simulink model "ground_state_ridgid"  (R2017b)
settings: Solver=VariableStepAuto  StartTime=0.0  StopTime=10  RelTol=1e-3
undefined symbols (not defined in the file or in its folder): refo
settings Model: Creator=benma  LastModifiedBy=benma

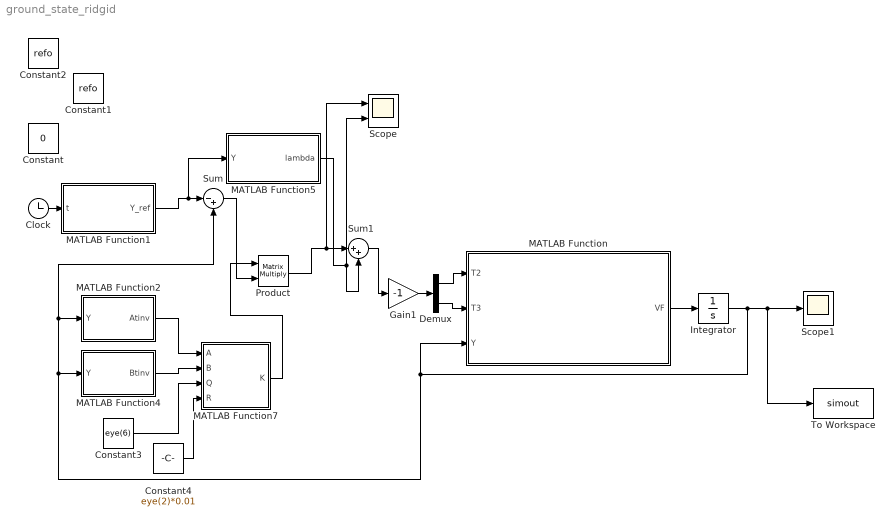
== system ground_state_ridgid ==
  Clock : Clock
  Constant : Constant  Value=0
  Constant1 : Constant  Value=refo
  Constant2 : Constant  Value=refo
  Constant3 : Constant  Value=eye(6)
  Constant4 : Constant  Value=eye(2)*0.01
  Demux : Demux  Outputs=2
  Gain1 : Gain  Gain=-1
  Integrator : Integrator  InitialCondition=refo
  MATLAB Function : MATLAB Function  TreatAsAtomicUnit=on
  MATLAB Function1 : MATLAB Function  TreatAsAtomicUnit=on
  MATLAB Function2 : MATLAB Function  TreatAsAtomicUnit=on
  MATLAB Function4 : MATLAB Function  TreatAsAtomicUnit=on
  MATLAB Function5 : MATLAB Function  TreatAsAtomicUnit=on
  MATLAB Function7 : MATLAB Function  TreatAsAtomicUnit=on
  Product : Product  Multiplication=Matrix(*)
  Scope : Scope  NumInputPorts=2
  Scope1 : Scope
  Sum : Sum  Inputs=|-+
  Sum1 : Sum  Inputs=|++
  To Workspace : ToWorkspace  VariableName=simout  SaveFormat=Timeseries  SampleTime=-1
  wires:
  MATLAB Function/1(VF) -> Integrator/1
  Gain1/1 -> Demux/1
  Demux/1 -> MATLAB Function/1(T2)
  Demux/2 -> MATLAB Function/2(T3)
  MATLAB Function5/1(lambda) -> Sum1/2, Scope/2
  Sum1/1 -> Gain1/1
  Clock/1 -> MATLAB Function1/1(t)
  MATLAB Function1/1(Y_ref) -> MATLAB Function5/1(Y), Sum/1
  Integrator/1 -> To Workspace/1, Scope1/1, MATLAB Function/3(Y), MATLAB Function4/1(Y), MATLAB Function2/1(Y), Sum/2
  MATLAB Function2/1(Atinv) -> MATLAB Function7/1(A)
  MATLAB Function4/1(Btinv) -> MATLAB Function7/2(B)
  Constant3/1 -> MATLAB Function7/3(Q)
  Constant4/1 -> MATLAB Function7/4(R)
  Product/1 -> Scope/1, Sum1/1
  Sum/1 -> Product/2
  MATLAB Function7/1(K) -> Product/1

== matlab function ground_state_ridgid/MATLAB Function ==
  data: T2 input; VF output; T3 input; Y input
function VF = threedof_ground(T2,T3,Y)
%THREEDOF_GROUND
%    VF = THREEDOF_GROUND(T2,T3,Y)

%    This function was generated by the Symbolic Math Toolbox version 8.0.
%    23-Nov-2018 17:29:58

t2 = Y(2);
t3 = t2.*2.0;
t4 = Y(3);
t5 = t4.*2.0;
t6 = Y(1);
t7 = Y(4);
t8 = t7.^2;
t9 = t2-t4;
t10 = sin(t9);
t11 = Y(5);
t12 = Y(6);
t13 = t2+t5;
t14 = sin(t13);
t15 = t11.^2;
t16 = cos(t5);
t17 = cos(t13);
t18 = t3+t5;
t19 = sin(t2);
t20 = t2+t4;
t21 = sin(t20);
t22 = t12.^2;
t23 = cos(t2);
t24 = cos(t3);
t25 = t24.*8.1e1;
t26 = t16.*4.5e1;
t27 = cos(t18);
t66 = t27.*9.0;
t28 = t25+t26-t66-1.69e2;
t29 = 1.0./t28;
t30 = cos(t6);
t31 = t3+t6;
t32 = cos(t31);
t33 = t32.*1.32435e4;
t34 = -t5+t6;
t35 = cos(t34);
t36 = t35.*4.4145e3;
t37 = t5+t6;
t38 = cos(t37);
t39 = t38.*4.4145e3;
t40 = t3+t5+t6;
t41 = cos(t40);
t42 = sin(t3);
t43 = sin(t5);
t44 = t8.*t10.*4.5e2;
t45 = t10.*t15.*4.5e2;
t46 = t10.*t22.*4.5e2;
t47 = t3+t4;
t48 = sin(t47);
t49 = cos(t9);
t50 = T3.*t17.*9.0e2;
t51 = sin(t18);
t52 = t15.*t19.*2.25e3;
t53 = sin(t4);
t54 = t8.*t21.*2.5e2;
t55 = t15.*t21.*2.5e2;
t56 = t21.*t22.*2.5e2;
t57 = cos(t20);
t58 = T3.*t57.*2.1e3;
t59 = t7.*t11.*t21.*5.0e2;
t60 = t7.*t12.*t21.*5.0e2;
t61 = t11.*t12.*t21.*5.0e2;
t62 = t7.*t10.*t11.*9.0e2;
t63 = t7.*t10.*t12.*9.0e2;
t64 = t10.*t11.*t12.*9.0e2;
t65 = t7.*t11.*t19.*4.5e3;
t67 = t2+t6;
t68 = cos(t67);
t69 = t68.*2.20725e4;
t70 = t2+t5+t6;
t71 = cos(t70);
t72 = -t2+t6;
t73 = cos(t72);
t74 = t2+t5-t6;
t75 = cos(t74);
t76 = t75.*4.4145e3;
t77 = t8.*t42.*1.35e3;
t78 = t15.*t42.*1.35e3;
t79 = t22.*t48.*4.5e2;
t80 = cos(t47);
t81 = T3.*t27.*9.0e2;
t82 = T2.*t23.*2.7e3;
t83 = cos(t4);
t84 = t7.*t11.*t42.*2.7e3;
t85 = t7.*t12.*t48.*9.0e2;
t86 = t11.*t12.*t48.*9.0e2;
VF = [t7;t11;t12;t29.*(T2.*2.3e3-t30.*3.1392e4+t33+t36+t39-t41.*1.4715e3+t44+t45+t46+t50+t52+t54+t55+t56+t58+t59+t60+t61+t62+t63+t64+t65+t77+t82-T2.*t16.*9.0e2-T2.*t17.*9.0e2-T3.*t23.*2.7e3-T3.*t49.*2.7e3-t8.*t14.*1.5e2+t8.*t19.*2.25e3-t14.*t15.*1.5e2-t8.*t51.*1.5e2-t7.*t11.*t14.*3.0e2).*(-3.0./5.0e1);t29.*(T2.*7.0e3-T3.*4.7e3-t30.*3.1392e4+t33+t36+t39-t41.*1.4715e3+t44+t45+t46+t50+t52+t54+t55+t56+t58+t59+t60+t61+t62+t63+t64+t65+t69-t71.*2.943e3-t73.*2.6487e4+t76+t78+t79+t81+t84+t85+t86-T2.*t16.*9.0e2-T2.*t17.*1.8e3+T2.*t23.*5.4e3-T3.*t23.*2.7e3-T2.*t27.*9.0e2-T3.*t49.*2.7e3+T3.*t80.*2.7e3-T3.*t83.*5.7e3-t8.*t14.*9.0e2+t8.*t19.*7.2e3-t14.*t15.*1.5e2+t8.*t42.*2.7e3-t8.*t43.*7.5e2+t8.*t48.*4.5e2-t15.*t43.*7.5e2-t8.*t51.*1.5e2-t8.*t53.*1.45e3+t15.*t48.*4.5e2-t15.*t53.*1.45e3-t22.*t53.*1.45e3-t7.*t11.*t14.*3.0e2-t7.*t11.*t43.*1.5e3+t7.*t11.*t48.*9.0e2-t7.*t11.*t53.*2.9e3-t7.*t12.*t53.*2.9e3-t11.*t12.*t53.*2.9e3).*(3.0./5.0e1);t29.*(T2.*4.7e3-T3.*1.9e4+t69-t71.*2.943e3-t73.*2.6487e4+t76+t77+t78+t79+t81+t82+t84+t85+t86-cos(t2+t4+t6).*2.4525e3+cos(t2+t4-t6).*5.886e3+cos(t2-t4+t6).*8.829e3-cos(-t2+t4+t6).*1.32435e4-T2.*t17.*9.0e2+T3.*t24.*8.1e3-T2.*t27.*9.0e2+T2.*t49.*2.7e3-T2.*t57.*2.1e3-T2.*t80.*2.7e3+T3.*t80.*5.4e3+T2.*t83.*5.7e3-T3.*t83.*1.14e4+t8.*t10.*2.25e3-t8.*t14.*7.5e2+t8.*t19.*4.95e3-t8.*t21.*8.5e2-t8.*t43.*1.5e3+t8.*t48.*9.0e2-t15.*t43.*1.5e3+t8.*t51.*1.5e2-t8.*t53.*5.0e3+t15.*t48.*9.0e2-t22.*t43.*7.5e2+t15.*t51.*1.5e2-t15.*t53.*5.0e3+t22.*t51.*1.5e2-t22.*t53.*1.45e3-t7.*t11.*t43.*3.0e3-t7.*t12.*t43.*1.5e3+t7.*t11.*t48.*1.8e3-t11.*t12.*t43.*1.5e3+t7.*t11.*t51.*3.0e2+t7.*t12.*t51.*3.0e2-t7.*t11.*t53.*1.0e4-t7.*t12.*t53.*2.9e3+t11.*t12.*t51.*3.0e2-t11.*t12.*t53.*2.9e3).*(-3.0./5.0e1)];

== matlab function ground_state_ridgid/MATLAB Function1 ==
  data: t input; Y_ref output
function Y_ref = Reference(t)
%REFERENCE
%    Y_REF = REFERENCE(T)

%    This function was generated by the Symbolic Math Toolbox version 8.0.
%    15-Dec-2018 14:08:43

t2 = t.^2;
t3 = exp(t2);
t4 = 1.0./t3.^(1.0./3.0);
t5 = exp(-2.5e1./3.0);
t6 = exp(t);
t7 = t6.^(1.0e1./3.0);
t8 = t4.*t5.*t7.*pi.*(1.0./2.0);
t9 = cos(t8);
t10 = sin(t8);
t11 = t-5.0;
t12 = t11.^2;
t26 = t12.*(1.0./3.0);
t13 = exp(-t26);
t14 = t9.*4.0;
t15 = t9.^2;
t16 = t10.^2;
t17 = t14+t15+t16+4.0;
t18 = sqrt(t17);
t19 = t10+t18;
t20 = t9+2.0;
t21 = 1.0./t20;
t22 = t4.*t5.*t6.^(1.0e1./3.0).*pi.*(5.0./3.0);
t25 = t.*t4.*t5.*t7.*pi.*(1.0./3.0);
t23 = t22-t25;
t24 = 1.0./t20.^2;
t27 = t.*(2.0./3.0);
t28 = t27-1.0e1./3.0;
t29 = t13.*t28.*pi.*(1.0./2.0);
Y_ref = [atan(t19.*t21).*2.0;t13.*pi.*(-1.0./2.0);t13.*pi.*(1.0./2.0);(t21.*(t9.*t23-t10.*1.0./sqrt(t17).*t23.*2.0).*2.0+t10.*t19.*t23.*t24.*2.0)./(t19.^2.*t24+1.0);t29;-t29];

== matlab function ground_state_ridgid/MATLAB Function2 ==
  data: Y input; Atinv output
function Atinv = LinA(Y)
%LINA
%    ATINV = LINA(Y)

%    This function was generated by the Symbolic Math Toolbox version 8.0.
%    15-Dec-2018 02:05:19

t2 = Y(2);
t3 = t2.*2.0;
t4 = Y(3);
t5 = t4.*2.0;
t6 = Y(1);
t7 = cos(t3);
t8 = t7.*8.1e1;
t9 = cos(t5);
t10 = t9.*4.5e1;
t11 = t3+t5;
t12 = cos(t11);
t152 = t12.*9.0;
t13 = t8+t10-t152-1.69e2;
t14 = 1.0./t13;
t15 = t3+t6;
t16 = sin(t15);
t17 = t3+t5+t6;
t18 = sin(t17);
t19 = Y(4);
t20 = t2-t4;
t21 = cos(t20);
t22 = Y(5);
t23 = t19.^2;
t24 = Y(6);
t25 = t2+t5;
t26 = cos(t25);
t27 = t22.^2;
t28 = cos(t2);
t29 = t2+t4;
t30 = cos(t29);
t31 = t24.^2;
t32 = sin(t5);
t33 = sin(t20);
t34 = t3+t4;
t35 = sin(t34);
t36 = sin(t25);
t37 = sin(t11);
t38 = sin(t4);
t39 = sin(t29);
t40 = sin(t2);
t41 = t28.*3.0;
t42 = cos(t4);
t43 = t30+t41+t42+4.0;
t44 = 1.0./t43;
t45 = cos(t6);
t46 = t2+t6;
t47 = cos(t46);
t48 = t4+t6;
t49 = cos(t48);
t50 = t2+t4-t6;
t51 = cos(t50);
t52 = t3+t4+t6;
t53 = cos(t52);
t54 = -t4+t6;
t55 = cos(t54);
t56 = cos(t17);
t57 = t56.*1.4715e3;
t58 = t2+t4+t6;
t59 = cos(t58);
t60 = sin(t3);
t61 = t23.*t37.*3.0e2;
t62 = t27.*t37.*1.5e2;
t63 = t31.*t37.*1.5e2;
t64 = t23.*t39.*3.3e3;
t65 = t19.*t22.*t37.*3.0e2;
t66 = t19.*t24.*t37.*3.0e2;
t67 = t22.*t24.*t37.*3.0e2;
t68 = t49.*1.4715e3;
t69 = t2-t4+t6;
t70 = cos(t69);
t71 = t53.*4.4145e3;
t72 = t2+t5+t6;
t73 = cos(t72);
t74 = t73.*1.4715e3;
t75 = t59.*9.81e3;
t76 = t23.*t32.*3.0e2;
t77 = t27.*t32.*3.0e2;
t78 = t31.*t32.*1.5e2;
t79 = t23.*t33.*9.0e2;
t80 = t23.*t35.*9.0e2;
t81 = t23.*t36.*6.0e2;
t82 = t27.*t35.*4.5e2;
t83 = t27.*t36.*4.5e2;
t84 = t31.*t36.*3.0e2;
t85 = t27.*t40.*4.5e2;
t86 = t23.*t38.*3.3e3;
t87 = t27.*t38.*1.95e3;
t88 = t31.*t38.*2.0e2;
t89 = t27.*t39.*1.55e3;
t90 = t31.*t39.*2.0e2;
t91 = t19.*t22.*t39.*3.1e3;
t92 = t19.*t24.*t39.*4.0e2;
t93 = t22.*t24.*t39.*4.0e2;
t94 = t19.*t22.*t32.*6.0e2;
t95 = t19.*t24.*t32.*3.0e2;
t96 = t22.*t24.*t32.*3.0e2;
t97 = t19.*t22.*t35.*9.0e2;
t98 = t19.*t22.*t36.*9.0e2;
t99 = t19.*t24.*t36.*6.0e2;
t100 = t22.*t24.*t36.*6.0e2;
t101 = t19.*t22.*t40.*9.0e2;
t102 = t19.*t22.*t38.*3.9e3;
t103 = t19.*t24.*t38.*4.0e2;
t104 = t22.*t24.*t38.*4.0e2;
t107 = t51.*7.3575e3;
t145 = t45.*8.3385e3;
t146 = t47.*4.4145e3;
t147 = t70.*4.4145e3;
t148 = t55.*1.1772e4;
t149 = t27.*t33.*4.5e2;
t150 = t19.*t22.*t33.*9.0e2;
t105 = t57+t61+t62+t63+t64+t65+t66+t67+t68+t71+t74+t75+t76+t77+t78-t79+t80+t81+t82+t83+t84+t85+t86+t87+t88+t89+t90+t91+t92+t93+t94+t95+t96+t97+t98+t99+t100+t101+t102+t103+t104-t107-t145-t146-t147-t148-t149-t150;
t106 = t47.*1.91295e4;
t108 = t53.*8.829e3;
t109 = -t2+t6;
t110 = cos(t109);
t111 = cos(t15);
t112 = t111.*1.32435e4;
t113 = t59.*6.3765e3;
t114 = t23.*t60.*2.7e3;
t115 = t27.*t60.*1.35e3;
t116 = t27.*t33.*9.0e2;
t117 = t23.*t35.*1.8e3;
t118 = t23.*t36.*3.0e2;
t119 = t31.*t33.*4.5e2;
t120 = t27.*t35.*9.0e2;
t121 = t27.*t36.*3.0e2;
t122 = t31.*t35.*4.5e2;
t123 = t31.*t36.*1.5e2;
t124 = t23.*t40.*7.5e3;
t125 = t27.*t40.*3.3e3;
t126 = t31.*t40.*4.5e2;
t127 = t27.*t39.*1.9e3;
t128 = t31.*t39.*5.5e2;
t129 = t19.*t22.*t39.*3.8e3;
t130 = t19.*t24.*t39.*1.1e3;
t131 = t22.*t24.*t39.*1.1e3;
t132 = t19.*t22.*t60.*2.7e3;
t133 = t19.*t22.*t33.*1.8e3;
t134 = t19.*t24.*t33.*9.0e2;
t135 = t19.*t22.*t35.*1.8e3;
t136 = t19.*t22.*t36.*6.0e2;
t137 = t22.*t24.*t33.*9.0e2;
t138 = t19.*t24.*t35.*9.0e2;
t139 = t19.*t24.*t36.*3.0e2;
t140 = t22.*t24.*t35.*9.0e2;
t141 = t22.*t24.*t36.*3.0e2;
t142 = t19.*t22.*t40.*6.6e3;
t143 = t19.*t24.*t40.*9.0e2;
t144 = t22.*t24.*t40.*9.0e2;
t155 = t45.*3.4335e4;
t156 = t49.*1.03005e4;
t157 = t110.*2.20725e4;
t158 = t55.*1.03005e4;
t159 = t31.*t38.*9.5e2;
t160 = t19.*t24.*t38.*1.9e3;
t161 = t22.*t24.*t38.*1.9e3;
t151 = t57+t61+t62+t63+t64+t65+t66+t67+t79+t106-t107+t108+t112+t113+t114+t115+t116+t117+t118+t119+t120+t121+t122+t123+t124+t125+t126+t127+t128+t129+t130+t131+t132+t133+t134+t135+t136+t137+t138+t139+t140+t141+t142+t143+t144-t155-t156-t157-t158-t159-t160-t161;
t153 = -t5+t6;
t154 = t5+t6;
t162 = sin(t153);
t163 = sin(t154);
t164 = t18.*2.943e3;
t165 = t21.*t23.*4.5e2;
t166 = t21.*t27.*4.5e2;
t167 = t21.*t31.*4.5e2;
t168 = t23.*t30.*2.5e2;
t169 = t27.*t30.*2.5e2;
t170 = t30.*t31.*2.5e2;
t171 = t19.*t22.*t30.*5.0e2;
t172 = t19.*t24.*t30.*5.0e2;
t173 = t22.*t24.*t30.*5.0e2;
t174 = t39.*t44.*t105.*(7.0./4.0);
t175 = t19.*t21.*t22.*9.0e2;
t176 = t19.*t21.*t24.*9.0e2;
t177 = t21.*t22.*t24.*9.0e2;
t178 = t37.*1.8e1;
t179 = 1.0./t13.^2;
t180 = cos(t153);
t181 = t180.*4.4145e3;
t182 = cos(t154);
t183 = t182.*4.4145e3;
t184 = t23.*t60.*1.35e3;
t185 = t23.*t33.*4.5e2;
t186 = t23.*t40.*2.25e3;
t187 = t27.*t40.*2.25e3;
t188 = t23.*t39.*2.5e2;
t189 = t27.*t39.*2.5e2;
t190 = t31.*t39.*2.5e2;
t191 = t9.*t44.*t151.*(3.0./4.0);
t192 = t19.*t22.*t39.*5.0e2;
t193 = t19.*t24.*t39.*5.0e2;
t194 = t22.*t24.*t39.*5.0e2;
t195 = t26.*t44.*t151.*(3.0./4.0);
t196 = t21.*t44.*t105.*(9.0./4.0);
t197 = t28.*t44.*t105.*(9.0./4.0);
t198 = t19.*t22.*t40.*4.5e3;
t228 = t45.*3.1392e4;
t229 = t27.*t36.*1.5e2;
t230 = t23.*t37.*1.5e2;
t231 = t26.*t44.*t105.*(3.0./4.0);
t232 = t19.*t22.*t36.*3.0e2;
t233 = t30.*t44.*t105.*(7.0./4.0);
t275 = t28.*t44.*t151.*(9.0./4.0);
t199 = -t57+t112+t119+t134+t137+t149+t150+t181+t183+t184+t185+t186+t187+t188+t189+t190+t191+t192+t193+t194+t195+t196+t197+t198-t228-t229-t230-t231-t232-t233-t275-t23.*t36.*1.5e2-t44.*t151.*(2.3e1./1.2e1);
t200 = t19.*t40.*4.5e3;
t201 = t22.*t40.*4.5e3;
t202 = t19.*t39.*5.0e2;
t203 = t22.*t39.*5.0e2;
t204 = t24.*t39.*5.0e2;
t205 = t19.*t33.*9.0e2;
t206 = t22.*t33.*9.0e2;
t207 = t24.*t33.*9.0e2;
t208 = sin(t6);
t209 = t16.*1.32435e4;
t210 = t162.*4.4145e3;
t211 = t163.*4.4145e3;
t212 = sin(t46);
t213 = sin(t72);
t214 = t213.*2.943e3;
t215 = sin(t109);
t216 = t215.*2.6487e4;
t217 = t2+t5-t6;
t218 = sin(t217);
t219 = t218.*4.4145e3;
t220 = cos(t34);
t221 = t12.*t23.*3.0e2;
t222 = t27.*t28.*2.25e3;
t223 = t36.*t44.*t151.*(3.0./2.0);
t224 = t36.*t44.*t105.*(3.0./4.0);
t225 = t19.*t22.*t28.*4.5e3;
t226 = t60.*1.62e2;
t227 = t178-t226;
t234 = t163.*8.829e3;
t235 = t26.*t27.*3.0e2;
t236 = t32.*t44.*t151.*(3.0./2.0);
t237 = t19.*t22.*t26.*6.0e2;
t238 = t37.*t44.*t105.*(3.0./2.0);
t239 = t32.*9.0e1;
t240 = t178-t239;
t241 = t47.*2.20725e4;
t242 = cos(t217);
t243 = t242.*4.4145e3;
t244 = t23.*t35.*4.5e2;
t245 = t23.*t40.*7.2e3;
t246 = t44.*t105.*(4.7e1./1.2e1);
t247 = t26.*t44.*t151.*(3.0./2.0);
t248 = t12.*t44.*t151.*(3.0./4.0);
t249 = t42.*t44.*t105.*(1.9e1./4.0);
t272 = t73.*2.943e3;
t273 = t110.*2.6487e4;
t274 = t31.*t38.*1.45e3;
t276 = t12.*t44.*t105.*(3.0./4.0);
t277 = t19.*t24.*t38.*2.9e3;
t278 = t22.*t24.*t38.*2.9e3;
t250 = -t57+t82+t97+t112+t114+t115+t119+t122+t132+t134+t137+t138+t140+t149+t150+t181+t183+t185+t187+t188+t189+t190+t191+t192+t193+t194+t196+t197+t198-t228-t229-t230-t231-t232-t233+t241+t243+t244+t245+t246+t247+t248+t249-t272-t273-t274-t276-t277-t278-t23.*t32.*7.5e2-t23.*t36.*9.0e2-t27.*t32.*7.5e2-t23.*t38.*1.45e3-t27.*t38.*1.45e3-t44.*t151.*(3.5e1./6.0)-t19.*t22.*t32.*1.5e3-t19.*t22.*t38.*2.9e3-t28.*t44.*t151.*(9.0./2.0)-t44.*t105.*t220.*(9.0./4.0);
t251 = t19.*t60.*2.7e3;
t252 = t22.*t60.*2.7e3;
t253 = t19.*t35.*9.0e2;
t254 = t22.*t35.*9.0e2;
t255 = t24.*t35.*9.0e2;
t256 = sin(t50);
t257 = t256.*5.886e3;
t258 = -t2+t4+t6;
t259 = sin(t258);
t260 = t259.*1.32435e4;
t261 = sin(t69);
t262 = sin(t58);
t263 = t262.*2.4525e3;
t264 = t31.*t220.*9.0e2;
t265 = t7.*t23.*2.7e3;
t266 = t7.*t27.*2.7e3;
t267 = t7.*t19.*t22.*5.4e3;
t268 = t19.*t24.*t220.*1.8e3;
t269 = t22.*t24.*t220.*1.8e3;
t270 = t37.*t44.*t151.*(3.0./2.0);
t271 = t40.*t44.*t151.*(9.0./4.0);
t279 = t218.*8.829e3;
t280 = t21.*t23.*2.25e3;
t281 = t23.*t220.*9.0e2;
t282 = t27.*t220.*9.0e2;
t283 = t12.*t27.*3.0e2;
t284 = t12.*t31.*3.0e2;
t285 = t31.*t42.*1.45e3;
t286 = t33.*t44.*t151.*(9.0./4.0);
t287 = t19.*t22.*t220.*1.8e3;
t288 = t35.*t44.*t105.*(9.0./2.0);
t289 = t12.*t19.*t22.*6.0e2;
t290 = t12.*t19.*t24.*6.0e2;
t291 = t12.*t22.*t24.*6.0e2;
t292 = t19.*t24.*t42.*2.9e3;
t293 = t22.*t24.*t42.*2.9e3;
t294 = t51.*5.886e3;
t295 = cos(t258);
t296 = t70.*8.829e3;
t297 = t23.*t33.*2.25e3;
t298 = t23.*t40.*4.95e3;
t299 = t44.*t105.*(9.5e1./6.0);
t300 = t44.*t151.*t220.*(9.0./4.0);
t301 = t30.*t44.*t151.*(7.0./4.0);
t302 = t42.*t44.*t105.*(1.9e1./2.0);
t303 = t59.*(-2.4525e3)+t62+t63+t65+t66+t67+t80+t115+t120+t122+t132+t135+t138+t140+t184+t195+t230+t241+t243+t248-t272-t273-t274-t275-t276-t277-t278+t294-t295.*1.32435e4+t296+t297+t298+t299+t300+t301+t302-t23.*t32.*1.5e3-t23.*t36.*7.5e2-t27.*t32.*1.5e3-t23.*t38.*5.0e3-t23.*t39.*8.5e2-t31.*t32.*7.5e2-t27.*t38.*5.0e3-t44.*t151.*(4.7e1./1.2e1)-t19.*t22.*t32.*3.0e3-t19.*t24.*t32.*1.5e3-t22.*t24.*t32.*1.5e3-t19.*t22.*t38.*1.0e4-t7.*t44.*t105.*(2.7e1./4.0)-t21.*t44.*t151.*(9.0./4.0)-t42.*t44.*t151.*(1.9e1./4.0)-t44.*t105.*t220.*(9.0./2.0);
t304 = t19.*t37.*3.0e2;
t305 = t22.*t37.*3.0e2;
t306 = t24.*t37.*3.0e2;
t307 = t19.*t35.*1.8e3;
t308 = t22.*t35.*1.8e3;
Atinv = reshape([0.0,0.0,0.0,t14.*(t18.*(-1.4715e3)-t208.*3.1392e4+t209+t210+t211).*(3.0./5.0e1),t14.*(t18.*1.4715e3+t208.*3.1392e4-t209-t210-t211-t212.*2.20725e4+t214+t216+t219).*(3.0./5.0e1),t14.*(t212.*(-2.20725e4)+t214+t216+t219+t257+t260-t261.*8.829e3+t263).*(-3.0./5.0e1),0.0,0.0,0.0,t14.*(t16.*-2.6487e4+t164+t165+t166+t167+t168+t169+t170+t171+t172+t173+t174+t175+t176+t177+t222+t224+t225+t265+t271-t12.*t23.*3.0e2-t23.*t26.*1.5e2+t23.*t28.*2.25e3-t26.*t27.*1.5e2-t19.*t22.*t26.*3.0e2-t33.*t44.*t105.*(9.0./4.0)-t40.*t44.*t105.*(9.0./4.0)-t36.*t44.*t151.*(3.0./4.0)).*(-3.0./5.0e1)+t179.*t199.*t227.*(3.0./5.0e1),t14.*(t16.*-2.6487e4+t164+t165+t166+t167+t168+t169+t170+t171+t172+t173+t174+t175+t176+t177-t212.*2.20725e4+t214-t216-t219-t221+t222-t223+t224+t225+t238+t264+t266+t267+t268+t269+t281+t282+t287+t288+t7.*t23.*5.4e3-t23.*t26.*9.0e2+t23.*t28.*7.2e3-t26.*t27.*1.5e2-t19.*t22.*t26.*3.0e2-t33.*t44.*t105.*(9.0./4.0)-t40.*t44.*t105.*(9.0./4.0)-t37.*t44.*t151.*(3.0./2.0)+t40.*t44.*t151.*(9.0./2.0)).*(3.0./5.0e1)-t179.*t227.*t250.*(3.0./5.0e1),t14.*(t212.*(-2.20725e4)+t214-t216-t219+t221+t238-t257-t260-t261.*8.829e3+t263+t264+t265+t266+t267+t268+t269-t270+t271+t280+t283+t284+t286+t289+t290+t291-t23.*t26.*7.5e2+t23.*t28.*4.95e3-t23.*t30.*8.5e2+t23.*t220.*1.8e3+t27.*t220.*1.8e3+t35.*t44.*t105.*9.0+t44.*t60.*t105.*(2.7e1./2.0)-t35.*t44.*t151.*(9.0./2.0)-t36.*t44.*t151.*(3.0./4.0)-t39.*t44.*t151.*(7.0./4.0)+t19.*t22.*t220.*3.6e3).*(-3.0./5.0e1)+t179.*t227.*t303.*(3.0./5.0e1),0.0,0.0,0.0,t14.*(t162.*-8.829e3-t164+t165+t166+t167-t168-t169-t170-t171-t172-t173-t174+t175+t176+t177+t221+t223+t234+t235+t236+t237+t23.*t26.*3.0e2-t33.*t44.*t105.*(9.0./4.0)-t36.*t44.*t105.*(3.0./2.0)).*(3.0./5.0e1)+t179.*t199.*t240.*(3.0./5.0e1),t14.*(t162.*-8.829e3-t164+t165+t166+t167-t168-t169-t170-t171-t172-t173-t174+t175+t176+t177-t213.*5.886e3+t221+t234+t235+t236+t237-t238+t270+t279+t285+t292+t293+t9.*t23.*1.5e3+t9.*t27.*1.5e3+t23.*t26.*1.8e3+t23.*t42.*1.45e3+t27.*t42.*1.45e3-t23.*t220.*4.5e2-t27.*t220.*4.5e2-t31.*t220.*4.5e2+t9.*t19.*t22.*3.0e3+t19.*t22.*t42.*2.9e3-t33.*t44.*t105.*(9.0./4.0)-t35.*t44.*t105.*(9.0./4.0)-t36.*t44.*t105.*(3.0./2.0)+t38.*t44.*t105.*(1.9e1./4.0)+t36.*t44.*t151.*3.0-t19.*t22.*t220.*9.0e2-t19.*t24.*t220.*9.0e2-t22.*t24.*t220.*9.0e2).*(-3.0./5.0e1)-t179.*t240.*t250.*(3.0./5.0e1),t14.*(t213.*-5.886e3-t221+t223-t238+t257-t260-t261.*8.829e3-t263+t270+t279+t280-t281-t282-t283-t284+t285+t286-t287-t288-t289-t290-t291+t292+t293+t9.*t23.*3.0e3+t9.*t27.*3.0e3+t9.*t31.*1.5e3+t23.*t26.*1.5e3+t23.*t30.*8.5e2+t23.*t42.*5.0e3+t27.*t42.*5.0e3-t31.*t220.*4.5e2+t9.*t19.*t22.*6.0e3+t9.*t19.*t24.*3.0e3+t9.*t22.*t24.*3.0e3+t19.*t22.*t42.*1.0e4+t38.*t44.*t105.*(1.9e1./2.0)+t35.*t44.*t151.*(9.0./4.0)-t38.*t44.*t151.*(1.9e1./4.0)+t39.*t44.*t151.*(7.0./4.0)-t19.*t24.*t220.*9.0e2-t22.*t24.*t220.*9.0e2).*(3.0./5.0e1)+t179.*t240.*t303.*(3.0./5.0e1),1.0,0.0,0.0,t14.*(t200+t201+t202+t203+t204+t205+t206+t207+t251-t19.*t36.*3.0e2-t19.*t37.*3.0e2-t22.*t36.*3.0e2).*(-3.0./5.0e1),t14.*(t201+t202+t203+t204+t205+t206+t207+t252+t253+t254+t255-t19.*t32.*1.5e3-t22.*t32.*1.5e3-t19.*t36.*1.8e3-t19.*t37.*3.0e2-t19.*t38.*2.9e3-t22.*t36.*3.0e2+t19.*t40.*1.44e4-t22.*t38.*2.9e3-t24.*t38.*2.9e3+t19.*t60.*5.4e3).*(3.0./5.0e1),t14.*(t251+t252+t255+t304+t305+t306+t307+t308-t19.*t32.*3.0e3+t19.*t33.*4.5e3-t22.*t32.*3.0e3-t19.*t36.*1.5e3-t24.*t32.*1.5e3-t19.*t38.*1.0e4-t19.*t39.*1.7e3+t19.*t40.*9.9e3-t22.*t38.*1.0e4-t24.*t38.*2.9e3).*(-3.0./5.0e1),0.0,1.0,0.0,t14.*(t200+t201+t202+t203+t204+t205+t206+t207-t19.*t36.*3.0e2-t22.*t36.*3.0e2).*(-3.0./5.0e1),t14.*(t200+t201+t202+t203+t204+t205+t206+t207+t251+t252+t253+t254+t255-t19.*t32.*1.5e3-t22.*t32.*1.5e3-t19.*t36.*3.0e2-t19.*t38.*2.9e3-t22.*t36.*3.0e2-t22.*t38.*2.9e3-t24.*t38.*2.9e3).*(3.0./5.0e1),t14.*(t251+t252+t255+t304+t305+t306+t307+t308-t19.*t32.*3.0e3-t22.*t32.*3.0e3-t24.*t32.*1.5e3-t19.*t38.*1.0e4-t22.*t38.*1.0e4-t24.*t38.*2.9e3).*(-3.0./5.0e1),0.0,0.0,1.0,t14.*(t202+t203+t204+t205+t206+t207).*(-3.0./5.0e1),t14.*(t202+t203+t204+t205+t206+t207+t253+t254+t255-t19.*t38.*2.9e3-t22.*t38.*2.9e3-t24.*t38.*2.9e3).*(3.0./5.0e1),t14.*(t253+t254+t255+t304+t305+t306-t19.*t32.*1.5e3-t22.*t32.*1.5e3-t24.*t32.*1.5e3-t19.*t38.*2.9e3-t22.*t38.*2.9e3-t24.*t38.*2.9e3).*(-3.0./5.0e1)],[6,6]);

== matlab function ground_state_ridgid/MATLAB Function5 ==
  data: Y input; lambda output
function lambda = ridgid_torque(Y)
%RIDGID_TORQUE
%    LAMBDA = RIDGID_TORQUE(Y)

%    This function was generated by the Symbolic Math Toolbox version 8.0.
%    24-Nov-2018 22:24:49

t2 = Y(2);
t3 = Y(3);
t4 = Y(1);
t5 = t2.*2.0;
t6 = Y(4);
t7 = sin(t5);
t8 = Y(5);
t9 = t6.^2;
t10 = t2-t3;
t11 = sin(t10);
t12 = t8.^2;
t13 = t3.*2.0;
t14 = Y(6);
t15 = t3+t5;
t16 = sin(t15);
t17 = t2+t13;
t18 = sin(t17);
t19 = t14.^2;
t20 = t5+t13;
t21 = sin(t20);
t22 = sin(t2);
t23 = t2+t3;
t24 = sin(t23);
t25 = sin(t3);
t26 = cos(t2);
t27 = t26.*3.0;
t28 = cos(t3);
t29 = cos(t23);
t30 = t27+t28+t29+4.0;
t31 = 1.0./t30;
t32 = cos(t4);
t33 = t2+t4;
t34 = cos(t33);
t35 = t3+t4;
t36 = cos(t35);
t37 = t2+t3-t4;
t38 = cos(t37);
t39 = t3+t4+t5;
t40 = cos(t39);
t41 = -t3+t4;
t42 = cos(t41);
t43 = t4+t5+t13;
t44 = cos(t43);
t45 = t44.*1.4715e3;
t46 = t2+t3+t4;
t47 = cos(t46);
t48 = sin(t13);
t49 = t9.*t11.*9.0e2;
t50 = t9.*t21.*3.0e2;
t51 = t12.*t21.*1.5e2;
t52 = t19.*t21.*1.5e2;
t53 = t9.*t24.*3.3e3;
t54 = t6.*t8.*t21.*3.0e2;
t55 = t6.*t14.*t21.*3.0e2;
t56 = t8.*t14.*t21.*3.0e2;
lambda = [t31.*(t32.*-3.4335e4+t34.*1.91295e4-t36.*1.03005e4-t38.*7.3575e3+t40.*8.829e3-t42.*1.03005e4+t45+t47.*6.3765e3+t49+t50+t51+t52+t53+t54+t55+t56-cos(-t2+t4).*2.20725e4+cos(t4+t5).*1.32435e4+t7.*t9.*2.7e3+t7.*t12.*1.35e3+t11.*t12.*9.0e2+t9.*t16.*1.8e3+t9.*t18.*3.0e2+t12.*t16.*9.0e2+t11.*t19.*4.5e2+t12.*t18.*3.0e2+t9.*t22.*7.5e3+t12.*t22.*3.3e3+t16.*t19.*4.5e2+t12.*t24.*1.9e3+t18.*t19.*1.5e2+t19.*t22.*4.5e2+t19.*t24.*5.5e2-t19.*t25.*9.5e2+t6.*t7.*t8.*2.7e3+t6.*t8.*t11.*1.8e3+t6.*t8.*t16.*1.8e3+t6.*t11.*t14.*9.0e2+t6.*t8.*t18.*6.0e2+t8.*t11.*t14.*9.0e2+t6.*t8.*t22.*6.6e3+t6.*t14.*t16.*9.0e2+t6.*t8.*t24.*3.8e3+t6.*t14.*t18.*3.0e2+t8.*t14.*t16.*9.0e2+t8.*t14.*t18.*3.0e2+t6.*t14.*t22.*9.0e2+t6.*t14.*t24.*1.1e3+t8.*t14.*t22.*9.0e2-t6.*t14.*t25.*1.9e3+t8.*t14.*t24.*1.1e3-t8.*t14.*t25.*1.9e3).*8.333333333333333e-4;t31.*(t32.*(-8.3385e3)-t34.*4.4145e3+t36.*1.4715e3-t38.*7.3575e3+t40.*4.4145e3-t42.*1.1772e4+t45+t47.*9.81e3-t49+t50+t51+t52+t53+t54+t55+t56+cos(t2+t4+t13).*1.4715e3-cos(t2-t3+t4).*4.4145e3-t11.*t12.*4.5e2+t9.*t16.*9.0e2+t9.*t18.*6.0e2+t12.*t16.*4.5e2+t12.*t18.*4.5e2+t9.*t25.*3.3e3+t12.*t22.*4.5e2+t12.*t24.*1.55e3+t12.*t25.*1.95e3+t18.*t19.*3.0e2+t19.*t24.*2.0e2+t19.*t25.*2.0e2+t9.*t48.*3.0e2+t12.*t48.*3.0e2+t19.*t48.*1.5e2-t6.*t8.*t11.*9.0e2+t6.*t8.*t16.*9.0e2+t6.*t8.*t18.*9.0e2+t6.*t8.*t22.*9.0e2+t6.*t8.*t24.*3.1e3+t6.*t14.*t18.*6.0e2+t6.*t8.*t25.*3.9e3+t8.*t14.*t18.*6.0e2+t6.*t14.*t24.*4.0e2+t6.*t14.*t25.*4.0e2+t8.*t14.*t24.*4.0e2+t8.*t14.*t25.*4.0e2+t6.*t8.*t48.*6.0e2+t6.*t14.*t48.*3.0e2+t8.*t14.*t48.*3.0e2).*8.333333333333333e-4];

== matlab function ground_state_ridgid/MATLAB Function4 ==
  data: Y input; Btinv output
function Btinv = LinB(Y)
%LINB
%    BTINV = LINB(Y)

%    This function was generated by the Symbolic Math Toolbox version 8.0.
%    15-Dec-2018 02:08:11

t2 = Y(2);
t3 = t2.*2.0;
t4 = Y(3);
t5 = t4.*2.0;
t6 = cos(t5);
t7 = cos(t2);
t8 = t2+t5;
t9 = cos(t8);
t10 = t9.*9.0e2;
t11 = cos(t3);
t12 = t11.*8.1e1;
t13 = t6.*4.5e1;
t14 = t3+t5;
t15 = cos(t14);
t18 = t15.*9.0;
t16 = t12+t13-t18-1.69e2;
t17 = 1.0./t16;
t19 = t6.*9.0e2;
t20 = t7.*2.7e3;
t21 = t2+t4;
t22 = cos(t21);
t23 = t22.*2.1e3;
t24 = t2-t4;
t25 = cos(t24);
t26 = t15.*9.0e2;
t27 = cos(t4);
t28 = t3+t4;
t29 = cos(t28);
t30 = t29.*2.7e3;
t31 = t17.*(t10-t20+t23-t25.*2.7e3+t26-t27.*5.7e3+t30-4.7e3).*(3.0./5.0e1);
Btinv = reshape([0.0,0.0,0.0,t17.*(t10+t19-t20-2.3e3).*(3.0./5.0e1),t17.*(t7.*-5.4e3+t9.*1.8e3+t19+t26-7.0e3).*(-3.0./5.0e1),t31,0.0,0.0,0.0,t17.*(t10-t20+t23-t25.*2.7e3).*(-3.0./5.0e1),t31,t17.*(t11.*8.1e3+t26-t27.*1.14e4+t29.*5.4e3-1.9e4).*(-3.0./5.0e1)],[6,2]);

== matlab function ground_state_ridgid/MATLAB Function7 ==
  data: A input; K output; B input; Q input; R input
function K = SDLQR(A,B,Q,R)
coder.extrinsic('ordschur')
H=[double(A) -double(B)*inv(R)*double(B.');
    -Q -double(A.')];
[n,m]=size(A);
[z,t] = schur(H,'real');
[z,t,Success] = ordschur(z,t,'lhp');
X1 = z(1:n,1:n);
X2 = z(n+1:n*2,1:n);
X=X2*inv(X1);
dB = double(B);
K = inv(R)*dB.'*X;
K=K
